simulink model "Plant"  (R2020b)
settings: Solver=VariableStepAuto  StartTime=0.0  StopTime=10.0  RelTol=1e-3
undefined symbols (not defined in the file): b, m
settings Model: DataDictionary=cruise_control_dd.sldd  Creator=ADMIN  LastModifiedBy=ADMIN
settings DataIOCC: SaveOutput=off  SaveTime=off

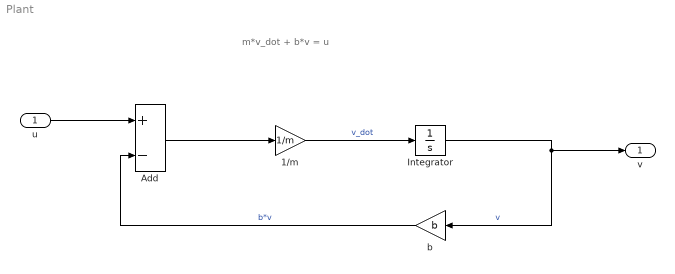
== system Plant ==
  note: m*v_dot + b*v = u
  u : Inport  OutDataTypeStr=double  PortDimensions=1
  1/m : Gain  Gain=1/m
  Add : Sum  Inputs=+-
  Integrator : Integrator
  b : Gain  Gain=b
  v : Outport  OutDataTypeStr=double  PortDimensions=1  SampleTime=0
  wires:
  Integrator/1 -> b/1, v/1  "v"
  1/m/1 -> Integrator/1  "v_dot"
  b/1 -> Add/2  "b*v"
  Add/1 -> 1/m/1
  u/1 -> Add/1
